simulink model "ThirdOrderCascadeSingleBitSC"  (R2021b)
settings: Solver=VariableStepDiscrete  StartTime=0.0  StopTime=(N-1)*Ts  RelTol=1e-3  EnableMultiTasking=on
undefined symbols (not defined in the file or in its folder): Ain, ao1, ao2, avnl1, avnl2, avnl3, avnl4, Cint1, Cint2, cload, cnl1, cnl2, cpar1, cpar2, Cs11, Cs12, Cs21, Cs22, f, FH, fin, FL, fs, gm1, gm2, innoise1, innoise2, io1, io2, M, N, osp, ron1, ron2, sinker, temp, Ts, vref
libraries: fesclib x3, quantrealib x2
settings Model: SimulationMode=accelerator  Creator=moreno  LastModifiedBy=jrosa
settings SolverCC: AlgebraicLoopSolver=TrustRegion
settings DataIOCC: LimitDataPoints=on  SaveFormat=Array  ReturnWorkspaceOutputs=off  SignalLoggingName=sigsOut
settings OptimizationCC: BooleanDataType=off  ExpressionDepthLimit=2147483647  LifeSpan=inf
settings DebuggingCC: SaveWithParameterizedLinksMsg=none  UnderspecifiedInitializationDetection=Classic  MergeDetectMultiDrivingBlocksExec=none  SignalResolutionControl=TryResolveAllWithWarning  MultiTaskDSMMsg=warning  MultiTaskCondExecSysMsg=none  FcnCallInpInsideContextMsg=warning  UnconnectedLineMsg=none  StateNameClashWarn=warning  SFUnexpectedBacktrackingDiag=warning  SFNoUnconditionalDefaultTransitionDiag=warning  SFExecutionAtInitializationDiag=none  SFMachineParentedDataDiag=warning  ArithmeticOperatorsInVariantConditions=warning
settings HardwareCC: ProdBitPerPointer=32  ProdBitPerSizeT=32  ProdBitPerPtrDiffT=32  ProdLargestAtomicFloat=None  ProdIntDivRoundTo=Undefined  ProdEndianess=Unspecified  ProdWordSize=32  ProdHWDeviceType=32-bit Generic  TargetUnknown=on
settings ModelReferenceCC: PropagateSignalLabelsOutOfModel=off
settings SFSimCC: SimUseLocalCustomCode=off  CustomCodeUndefinedFunction=UseInterfaceOnly
settings RTWCC: RTWUseLocalCustomCode=off
settings CodeAppCC: StateflowObjectComments=on
settings GRTTargetCC: TargetLangStandard=C89/C90 (ANSI)  CombineOutputUpdateFcns=off  GRTInterface=on
settings ConfigComp: CovMetricSettings=dw  CovSaveCumulativeToWorkspaceVar=on  CovSaveSingleToWorkspaceVar=on  CovExternalEMLEnable=off

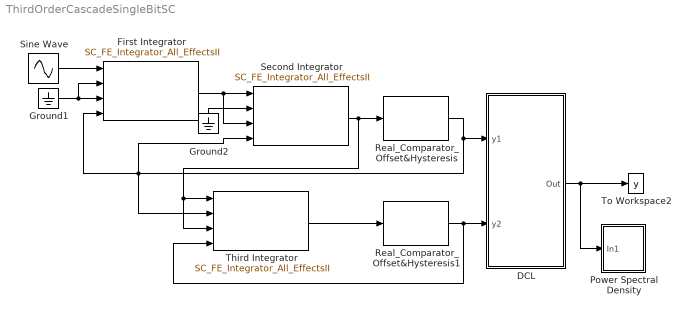
== system ThirdOrderCascadeSingleBitSC ==
  DCL : Subsystem
      mask Display: disp(strvcat('Cancelation','  Logic'))
  First Integrator : fesclib/SC_FE_Integrator_All_EffectsII  c=[Cint1,Cs11,Cs21,cnl1,cnl2]  var=[0,innoise1,temp,ron1]  ops=[osp,-osp]  ao=[ao1,gm1,io1]  avnl=[avnl1,avnl2,avnl3,avnl4]  cp=[cpar1,cpar2,cload]  phi=phi1  ts=Ts  settlingon=on  setin=on  idown=a  idnext=b
      link override C11: Value=6e-12
      link override C12: Value=6e-12
      link override From: GotoTag=b
      link override Goto: GotoTag=a
  Ground1 : Ground
  Ground2 : Ground
  Power Spectral Density : Subsystem  AncestorBlock=SDtoolbox/Power Spectral Density  mask{SN=2, Fs=fs, fBL=1, fBH=fs/M, Fin=fin, N=N, Ntransient=0, VW=off, savename=savemat, Scale_type=linear}
      mask prompts: SN "Scope Number"; Fs "Sampling Frequency [Hz]"; fBL "Lower Band Bound [Hz]"; fBH "Upper Band Bound [Hz]"; Fin "Signal Frequency [Hz]"; N "Number of FFT Points"; Ntransient "Number of Transient Points"; VW "Variables Available in the Workspace"; savename "Nome of .mat File"; Scale_type "Scale"
      mask help: Calculates power spectral density, signal-to-noise ratio and effective number of bits of the Sigma-Delta modulator output
      mask init:
      | [f,FL,FH]=sinker_ini(Fs,fBL,fBH,Fin,N,SN);
      mask Help: web('PSD.html','-helpbrowser')
      mask Callback VW:
      | opt1=(get_param(gcb,'VW'));
      | switch opt1
      | 	case 'off'
      | 				set_param(gcb,'MaskEnables',{'on','on','on','on','on','on','on','on','off','on'});
      | 	case 'on'
      | 				set_param(gcb,'MaskEnables',{'on','on','on','on','on','on','on','on','on','on'});
      | end
      mask TypeOptions Scale_type: linear | logarithmic
      mask Display:
      | plot(0,0,1,1,[.14,.91,.91,.14,.14],[.86,.86,.40,.40,.86],[.85,.82,.80,.79,.75,.67,.63,.60,.57,.53,.41,.36,.33,.27,.24],[.49,.50,.53,.50,.49,.51,.54,.63,.54,.50,.50,.52,.82,.52,.45])
      | text(.54,.18, 'PSD','horizontalAlignment', 'center')
  Real_Comparator_Offset&Hysteresis : quantrealib/Real_Comparator_Offset&Hysteresis  Vhigh=vref  Vlow=-vref  OFFSET_PARAM=0  FLAG_PARAM=Without Hysteresys  H_PARAM=hys  phi=phi1  ts=Ts  qid=quant1
      link override Goto: GotoTag=quant1
  Real_Comparator_Offset&Hysteresis1 : quantrealib/Real_Comparator_Offset&Hysteresis  Vhigh=vref  Vlow=-vref  OFFSET_PARAM=0  FLAG_PARAM=Without Hysteresys  H_PARAM=hys  phi=phi1  ts=Ts  qid=quant2
      link override Goto: GotoTag=quant2
  Second Integrator : fesclib/SC_FE_Integrator_All_EffectsII  c=[Cint2,Cs12,Cs22,cnl1,cnl2]  var=[0,innoise2,temp,ron2]  ops=[osp,-osp]  ao=[ao2,gm2,io2]  avnl=[avnl1,avnl2,avnl3,avnl4]  cp=[cpar1,cpar2,cload]  phi=phi1  ts=Ts  settlingon=on  setin=on  idown=b  idnext=c
      link override C11: Value=1.5e-12
      link override C12: Value=1.5e-12
      link override From: GotoTag=c
      link override Goto: GotoTag=b
  Sine Wave : Sin  Amplitude=10^(Ain/20)  Frequency=2*pi*fin  SampleTime=0
  Third Integrator : fesclib/SC_FE_Integrator_All_EffectsII  c=[Cint2,Cs12,Cs22,cnl1,cnl2]  var=[0,innoise2,temp,ron2]  ops=[osp,-osp]  ao=[ao2,gm2,io2]  avnl=[avnl1,avnl2,avnl3,avnl4]  cp=[cpar1,cpar2,cload]  phi=phi1  ts=Ts  settlingon=on  setin=off  idown=c  idnext=c
      link override C11: Value=1.5e-12
      link override C12: Value=1.5e-12
      link override From: GotoTag=c
      link override Goto: GotoTag=c
  To Workspace2 : ToWorkspace  VariableName=y  SampleTime=Ts
      settings: MaxDataPoints=N
  wires:
  Sine Wave/1 -> First Integrator/1
  First Integrator/1 -> Second Integrator/3, Second Integrator/1
  Second Integrator/1 -> Real_Comparator_Offset&Hysteresis/1, Third Integrator/3, Third Integrator/1
  Real_Comparator_Offset&Hysteresis/1 -> DCL/1(y1), Third Integrator/2, First Integrator/4, Second Integrator/4
  Third Integrator/1 -> Real_Comparator_Offset&Hysteresis1/1
  Real_Comparator_Offset&Hysteresis1/1 -> DCL/2(y2), Third Integrator/4
  Ground2/1 -> Second Integrator/2
  DCL/1(Out) -> To Workspace2/1, Power Spectral Density/1(In1)
  Ground1/1 -> First Integrator/3, First Integrator/2

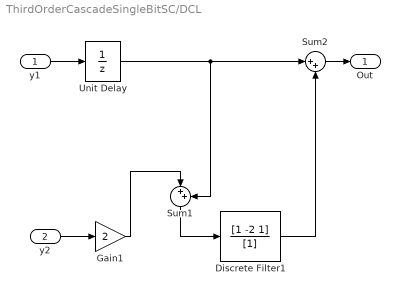
== system ThirdOrderCascadeSingleBitSC/DCL ==
  y1 : Inport
  y2 : Inport  Port=2
  Discrete Filter1 : DiscreteFilter  Numerator=[1 -2 1]  Denominator=[1]  SampleTime=Ts
  Gain1 : Gain  Gain=2  SaturateOnIntegerOverflow=on  OutDataTypeStr=Inherit: Same as input  ParamDataTypeStr=Inherit: Same as input
  Sum1 : Sum  Inputs=|++  InputSameDT=on  SaturateOnIntegerOverflow=on  OutDataTypeStr=Inherit: Same as first input
  Sum2 : Sum  Inputs=|++  InputSameDT=on  SaturateOnIntegerOverflow=on  OutDataTypeStr=Inherit: Same as first input
  Unit Delay : UnitDelay  SampleTime=Ts  HasFrameUpgradeWarning=on
  Out : Outport
  wires:
  Unit Delay/1 -> Sum2/1, Sum1/2
  Discrete Filter1/1 -> Sum2/2
  Gain1/1 -> Sum1/1
  Sum1/1 -> Discrete Filter1/1
  y1/1 -> Unit Delay/1
  y2/1 -> Gain1/1
  Sum2/1 -> Out/1

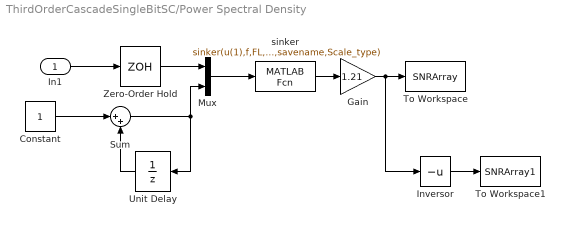
== system ThirdOrderCascadeSingleBitSC/Power Spectral Density ==
  In1 : Inport
  Constant : Constant
  Gain : Gain  Gain=1.21
  Inversor : UnaryMinus
  Mux : Mux  Inputs=2
  Sum : Sum  Inputs=|++  SaturateOnIntegerOverflow=on
  To Workspace : ToWorkspace  VariableName=SNRArray  SampleTime=-1
      settings: MaxDataPoints=1
  To Workspace1 : ToWorkspace  VariableName=SNRArray1  SampleTime=-1
      settings: MaxDataPoints=1
  Unit Delay : UnitDelay  SampleTime=1/Fs  HasFrameUpgradeWarning=on
  Zero-Order Hold : ZeroOrderHold  SampleTime=1/Fs
  sinker : MATLABFcn  MATLABFcn=sinker(u(1),f,FL,FH,N,Ntransient,u(2),SN,Fs,VW,savename,Scale_type)
  wires:
  Zero-Order Hold/1 -> Mux/1
  In1/1 -> Zero-Order Hold/1
  Mux/1 -> sinker/1
  Sum/1 -> Mux/2, Unit Delay/1
  Constant/1 -> Sum/1
  Unit Delay/1 -> Sum/2
  sinker/1 -> Gain/1
  Inversor/1 -> To Workspace1/1
  Gain/1 -> To Workspace/1, Inversor/1
